simulink model "UnDBlimp"  (R2021a)
settings: Solver=VariableStepAuto  StartTime=ti  StopTime=tf  RelTol=1e-3
values from neighbouring files (symbols this model uses):
  A_Obs = A    [ObserverDesign.m]
  A_real = A    [ObserverDesign.m]    (also in PreComputeForSimuUnDBlimp.m)
  B_Obs = [Bb11 L]    [ObserverDesign.m]
  B_real = B    [ObserverDesign.m]    (also in PreComputeForSimuUnDBlimp.m)
  C_Obs = eye(2)    [ObserverDesign.m]
  Cx_nominal = eye(2)    [ObserverDesign.m]    (also in PreComputeForSimuUnDBlimp.m)
  D_Obs = [0 0;0 0]    [ObserverDesign.m]
  D_real = [0;0]    [ObserverDesign.m]    (also in PreComputeForSimuUnDBlimp.m)
  G = -1/(C*(A-B*K)^(-1)*B)    [ObserverDesign.m]    (also in PreComputeForSimuUnDBlimp.m)
  K = place(A,B,Controller.poles)    [ObserverDesign.m]    (also in PreComputeForSimuUnDBlimp.m)
  zc = 10    [ObserverDesign.m]    (also in PreComputeForSimuUnDBlimp.m)
undefined symbols (not defined in the file or in its folder): IC, Noise, Observer
libraries: simulink x1
settings Model: Creator=perruquetti  LastModifiedBy=perruquetti
settings SolverCC: AlgebraicLoopSolver=TrustRegion
settings DataIOCC: ReturnWorkspaceOutputs=off
settings DebuggingCC: SFMachineParentedDataDiag=warning  ArithmeticOperatorsInVariantConditions=warning
settings SFSimCC: SimUseLocalCustomCode=off  CustomCodeUndefinedFunction=UseInterfaceOnly
settings RTWCC: RTWUseLocalCustomCode=off

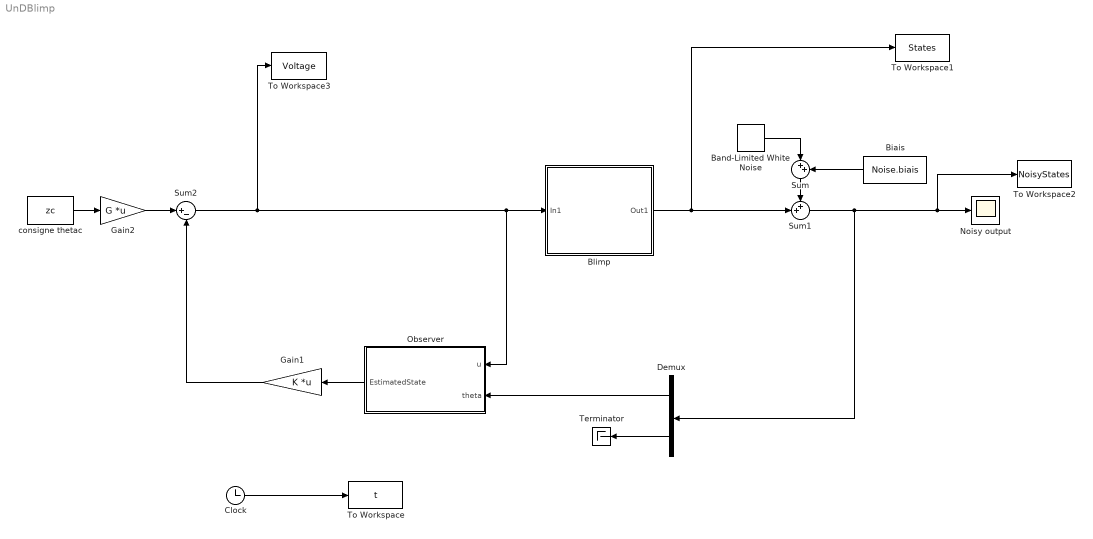
== system UnDBlimp ==
  Band-Limited White Noise : simulink/Sources/Band-Limited White Noise  Cov=Noise.power  Ts=Noise.sampling  seed=Noise.seed
  Biais : Constant  Value=Noise.biais
  Blimp : Subsystem
  Clock : Clock
  Demux : Demux  Outputs=2
  Gain1 : Gain  Gain=K  Multiplication=Matrix(K*u)
  Gain2 : Gain  Gain=G  Multiplication=Matrix(K*u)
  Noisy output : Scope
  Observer : Subsystem
  Sum : Sum  Inputs=|++
  Sum1 : Sum  Inputs=++|
  Sum2 : Sum  Inputs=|+-
  Terminator : Terminator
  To Workspace : ToWorkspace  VariableName=t  SampleTime=-1
  To Workspace1 : ToWorkspace  VariableName=States  SampleTime=-1
  To Workspace2 : ToWorkspace  VariableName=NoisyStates  SampleTime=-1
  To Workspace3 : ToWorkspace  VariableName=Voltage  SampleTime=-1
  consigne thetac : Constant  Value=zc
  wires:
  Band-Limited White Noise/1 -> Sum/1
  Biais/1 -> Sum/2
  Sum/1 -> Sum1/1
  Clock/1 -> To Workspace/1
  Blimp/1(Out1) -> Sum1/2, To Workspace1/1
  consigne thetac/1 -> Gain2/1
  Gain2/1 -> Sum2/1
  Gain1/1 -> Sum2/2
  Demux/1 -> Observer/2(theta)
  Sum2/1 -> Observer/1(u), Blimp/1(In1), To Workspace3/1
  Sum1/1 -> Demux/1, To Workspace2/1, Noisy output/1
  Demux/2 -> Terminator/1
  Observer/1(EstimatedState) -> Gain1/1

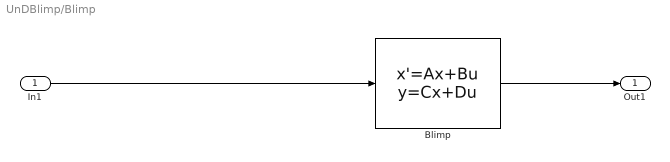
== system UnDBlimp/Blimp ==
  In1 : Inport
  Blimp : StateSpace  A=A_real  B=B_real  C=Cx_nominal  D=D_real  InitialCondition=IC.state
  Out1 : Outport  VectorParamsAs1DForOutWhenUnconnected=off
  wires:
  Blimp/1 -> Out1/1
  In1/1 -> Blimp/1

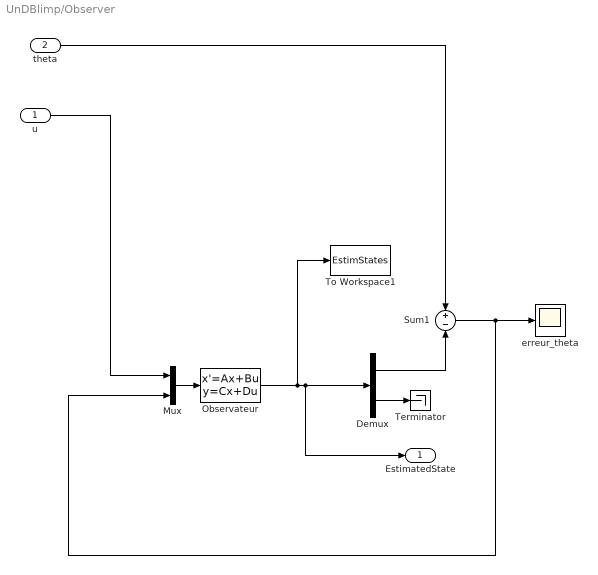
== system UnDBlimp/Observer ==
  u : Inport
  theta : Inport  Port=2
  Demux : Demux  Outputs=2
  Mux : Mux  Inputs=2
  Observateur : StateSpace  A=A_Obs  B=B_Obs  C=C_Obs  D=D_Obs  InitialCondition=Observer.IC
  Sum1 : Sum  Inputs=+-
  Terminator : Terminator
  To Workspace1 : ToWorkspace  VariableName=EstimStates  SampleTime=-1
  erreur_theta : Scope
  EstimatedState : Outport  VectorParamsAs1DForOutWhenUnconnected=off
  wires:
  theta/1 -> Sum1/1
  Demux/1 -> Sum1/2
  Sum1/1 -> Mux/2, erreur_theta/1
  Observateur/1 -> To Workspace1/1, EstimatedState/1, Demux/1
  Mux/1 -> Observateur/1
  Demux/2 -> Terminator/1
  u/1 -> Mux/1
